simulink model "amr_milestone01"  (R2025b)
settings: Solver=FixedStepDiscrete  StartTime=0.0  StopTime=12  FixedStep=0.01  RelTol=1e-3
undefined symbols (not defined in the file): DiscIntNeverNeededParam
settings Model: Creator=leeyj  LastModifiedBy=leeyj

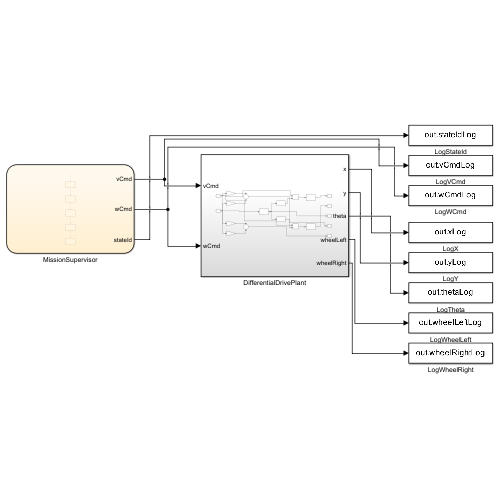
[thumbnail: Simulink's stored preview of the top-level diagram]
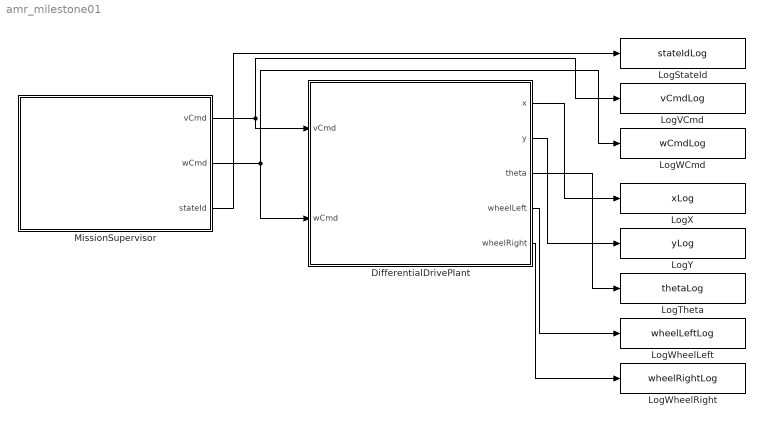
== system amr_milestone01 ==
  DifferentialDrivePlant : Subsystem
  LogStateId : ToWorkspace  VariableName=stateIdLog  SaveFormat=Timeseries  SampleTime=-1
  LogTheta : ToWorkspace  VariableName=thetaLog  SaveFormat=Timeseries  SampleTime=-1
  LogVCmd : ToWorkspace  VariableName=vCmdLog  SaveFormat=Timeseries  SampleTime=-1
  LogWCmd : ToWorkspace  VariableName=wCmdLog  SaveFormat=Timeseries  SampleTime=-1
  LogWheelLeft : ToWorkspace  VariableName=wheelLeftLog  SaveFormat=Timeseries  SampleTime=-1
  LogWheelRight : ToWorkspace  VariableName=wheelRightLog  SaveFormat=Timeseries  SampleTime=-1
  LogX : ToWorkspace  VariableName=xLog  SaveFormat=Timeseries  SampleTime=-1
  LogY : ToWorkspace  VariableName=yLog  SaveFormat=Timeseries  SampleTime=-1
  MissionSupervisor : Stateflow chart  TreatAsAtomicUnit=on
  wires:
  MissionSupervisor/1(vCmd) -> DifferentialDrivePlant/1(vCmd), LogVCmd/1
  MissionSupervisor/2(wCmd) -> DifferentialDrivePlant/2(wCmd), LogWCmd/1
  MissionSupervisor/3(stateId) -> LogStateId/1
  DifferentialDrivePlant/1(x) -> LogX/1
  DifferentialDrivePlant/2(y) -> LogY/1
  DifferentialDrivePlant/3(theta) -> LogTheta/1
  DifferentialDrivePlant/4(wheelLeft) -> LogWheelLeft/1
  DifferentialDrivePlant/5(wheelRight) -> LogWheelRight/1

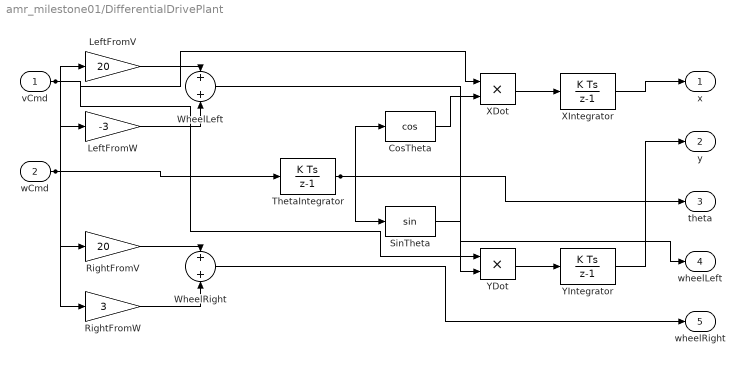
== system amr_milestone01/DifferentialDrivePlant ==
  vCmd : Inport
  wCmd : Inport  Port=2
  CosTheta : Trigonometry  Operator=cos
  LeftFromV : Gain  Gain=20
  LeftFromW : Gain  Gain=-3
  RightFromV : Gain  Gain=20
  RightFromW : Gain  Gain=3
  SinTheta : Trigonometry
  ThetaIntegrator : DiscreteIntegrator  gainval=1  SampleTime=0.01  ICPrevOutput=DiscIntNeverNeededParam  ICPrevScaledInput=DiscIntNeverNeededParam
  WheelLeft : Sum
  WheelRight : Sum
  XDot : Product  Inputs=**
  XIntegrator : DiscreteIntegrator  gainval=1  SampleTime=0.01  ICPrevOutput=DiscIntNeverNeededParam  ICPrevScaledInput=DiscIntNeverNeededParam
  YDot : Product  Inputs=**
  YIntegrator : DiscreteIntegrator  gainval=1  SampleTime=0.01  ICPrevOutput=DiscIntNeverNeededParam  ICPrevScaledInput=DiscIntNeverNeededParam
  x : Outport
  y : Outport  Port=2
  theta : Outport  Port=3
  wheelLeft : Outport  Port=4
  wheelRight : Outport  Port=5
  wires:
  vCmd/1 -> LeftFromV/1, RightFromV/1, XDot/1, YDot/1
  wCmd/1 -> LeftFromW/1, RightFromW/1, ThetaIntegrator/1
  LeftFromV/1 -> WheelLeft/1
  LeftFromW/1 -> WheelLeft/2
  RightFromV/1 -> WheelRight/1
  RightFromW/1 -> WheelRight/2
  ThetaIntegrator/1 -> CosTheta/1, SinTheta/1, theta/1
  CosTheta/1 -> XDot/2
  SinTheta/1 -> YDot/2
  XDot/1 -> XIntegrator/1
  YDot/1 -> YIntegrator/1
  XIntegrator/1 -> x/1
  YIntegrator/1 -> y/1
  WheelLeft/1 -> wheelLeft/1
  WheelRight/1 -> wheelRight/1

== stateflow chart amr_milestone01/MissionSupervisor ==
  state Initializing
    entry, during:
    vCmd = 0;
    wCmd = 0;
    stateId = uint8(0);
  state DriveStraight1
    entry, during:
    vCmd = 0.5;
    wCmd = 0;
    stateId = uint8(1);
  state TurnLeft
    entry, during:
    vCmd = 0;
    wCmd = pi/4;
    stateId = uint8(2);
  state DriveStraight2
    entry, during:
    vCmd = 0.5;
    wCmd = 0;
    stateId = uint8(3);
  state Stopped
    entry, during:
    vCmd = 0;
    wCmd = 0;
    stateId = uint8(4);
  (default) -> Initializing
  Initializing -> DriveStraight1 : after(1,sec)
  DriveStraight1 -> TurnLeft : after(4,sec)
  TurnLeft -> DriveStraight2 : after(2,sec)
  DriveStraight2 -> Stopped : after(4,sec)
  data: vCmd output double; wCmd output double; stateId output uint8
